simulink model "zumo_target"  (R2014a)
settings: Solver=ode3  SolverMode=SingleTasking  StartTime=0.0  StopTime=10  RelTol=1e-3
model workspace (MAT data in the model file):
  axleLength = Simulink.Parameter
  axleLength.Value = 9.5
  axleLength.Description = 'Distance between tire contact points
    | of the two wheels/treads
    | in units of centimeters.'
  axleLength.DataType = 'auto'
  commandPercmPerSecond = Simulink.Parameter
  commandPercmPerSecond.Value = 3.9547
  commandPercmPerSecond.Description = 'Convert units of ''command'' 
    | to units of ''cm/s''.
    | 
    | ''command'' is a value in the range [-256, 255].'
  commandPercmPerSecond.DataType = 'auto'
  symmetrizeMotors = Simulink.Parameter
  symmetrizeMotors.Value = 1
  symmetrizeMotors.Description = 'Scale one of the motor commands down 
    | (not up) to balance the motors. 
    | Once balanced, a value of x sent to either
    | motor will produce the same rate of rotation
    | in both motors.'
  symmetrizeMotors.DataType = 'auto'
  sampleTime = Simulink.Parameter
  sampleTime.Value = 0.01
  sampleTime.Description = 'Sample time (in seconds) of the trajectory simulator.'
  sampleTime.DataType = 'auto'
  commandThreshold = Simulink.Parameter
  commandThreshold.Value = 31.875
  commandThreshold.DataType = 'auto'
  plotRange = Simulink.Parameter
  plotRange.Value = 50
  plotRange.Description = 'Range of trajectory plot in units
    | of centimeters.'
  plotRange.DataType = 'auto'
undefined symbols (not defined in the file or in its folder): DiscIntNeverNeededParam
libraries: arduinolib x1, simulink x1, ZumoBotLib x1
settings Model: ExtModeTrigDuration=2  Creator=nrattner  LastModifiedBy=sandip
settings OptimizationCC: OptimizeModelRefInitCode=on  LifeSpan=1
settings DebuggingCC: UnderspecifiedInitializationDetection=Classic  SolverPrmCheckMsg=none
settings HardwareCC: ProdBitPerInt=16  ProdBitPerPointer=8  ProdIntDivRoundTo=Zero  ProdEndianess=LittleEndian  ProdWordSize=8  ProdHWDeviceType=Atmel->AVR
settings RTWCC: SystemTargetFile=realtime.tlc  GenerateMakefile=off  TemplateMakefile=realtime.tmf  Description=Run on Target Hardware  RTWVerbose=off  ProcessScript=realtime_make_rtw_hook
settings STFCustomTargetCC: TargetLibSuffix=.a  GenerateSampleERTMain=on  ConcurrentExecutionCompliant=off  GeneratePreprocessorConditionals=Use local settings  ERTCustomFileBanners=on  SupportNonInlinedSFcns=off  SupportVariableSizeSignals=on  MATLABClassNameForMDSCustomization=Simulink.SoftwareTarget.ERTCustomization  GRTInterface=off  SystemTargetFile=realtime.tlc
settings ERTTargetCC: CombineOutputUpdateFcns=off  SupportContinuousTime=on  SupportVariableSizeSignals=on  ExtModeTransport=3  ExtModeMexFile=ext_serial_win32_comm  ExtModeMexArgs=0 1 9600  ERTSrcFileBannerTemplate=realtime_code_template.cgt  ERTHdrFileBannerTemplate=realtime_code_template.cgt  ERTDataSrcFileTemplate=realtime_code_template.cgt  ERTDataHdrFileTemplate=realtime_code_template.cgt  ERTCustomFileTemplate=realtime_file_process.tlc

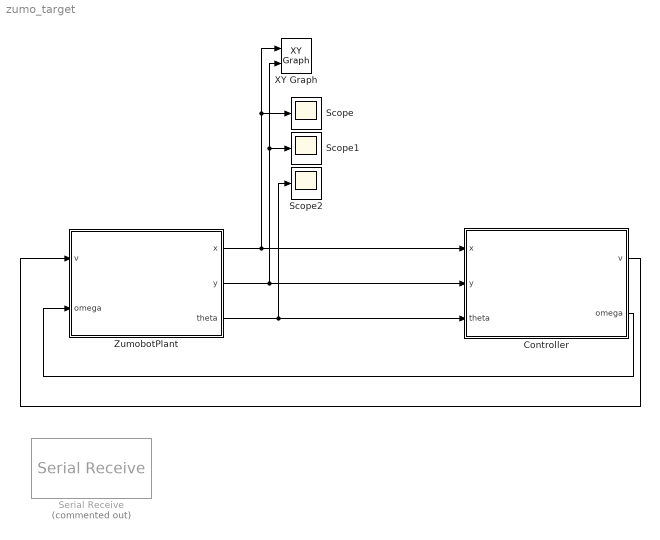
== system zumo_target ==
  Controller : Subsystem
  Scope : Scope
      settings: YMin=-0.000967084  YMax=-0.000967084
  Scope1 : Scope
      settings: YMin=0.0106562  YMax=0.0106562
  Scope2 : Scope
      settings: YMin=1.6613  YMax=1.6613  SaveName=ScopeData2
  Serial Receive : arduinolib/Serial Receive  Commented=on  portNumber=0  showOutStatus=on  sampleTime=1e-3
  XY Graph : simulink/Sinks/XY Graph  xmin=-10  xmax=10  ymin=-10  ymax=10  st=-1
  ZumobotPlant : Subsystem  Variant=on
  wires:
  ZumobotPlant/1(x) -> XY Graph/1, Scope/1, Controller/1(x)
  ZumobotPlant/2(y) -> Controller/2(y), XY Graph/2, Scope1/1
  ZumobotPlant/3(theta) -> Controller/3(theta), Scope2/1
  Controller/1(v) -> ZumobotPlant/1(v)
  Controller/2(omega) -> ZumobotPlant/2(omega)

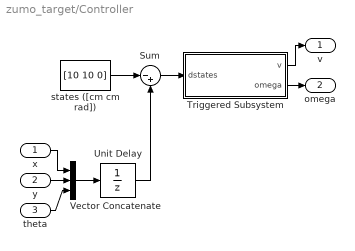
== system zumo_target/Controller ==
  x : Inport
  y : Inport  Port=2
  theta : Inport  Port=3
  Sum : Sum  Inputs=|-+
  Triggered Subsystem : Subsystem  TreatAsAtomicUnit=on
  Unit Delay : UnitDelay  SampleTime=-1
  Vector Concatenate : Concatenate  NumInputs=3
  states ([cm cm rad]) : Constant  Value=[10 10 0]
  v : Outport
  omega : Outport  Port=2
  wires:
  Unit Delay/1 -> Sum/2
  Vector Concatenate/1 -> Unit Delay/1
  Sum/1 -> Triggered Subsystem/1(dstates)
  states ([cm cm rad])/1 -> Sum/1
  Triggered Subsystem/1(v) -> v/1
  Triggered Subsystem/2(omega) -> omega/1
  y/1 -> Vector Concatenate/2
  theta/1 -> Vector Concatenate/3
  x/1 -> Vector Concatenate/1

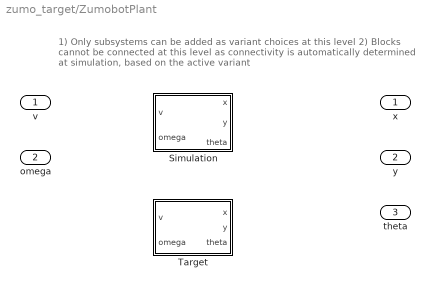
== system zumo_target/ZumobotPlant ==
  note: 1) Only subsystems can be added as variant choices at this level
      | 2) Blocks cannot be connected at this level as connectivity is
      | automatically determined at simulation, based on the active variant
  v : Inport
  omega : Inport  Port=2
  Simulation : Subsystem  VariantControl=sim==1
  Target : Subsystem  VariantControl=sim==0
  x : Outport
  y : Outport  Port=2
  theta : Outport  Port=3

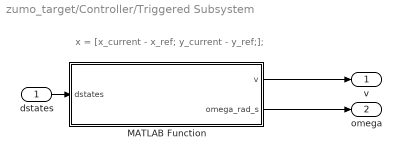
== system zumo_target/Controller/Triggered Subsystem ==
  note: x = [x_current - x_ref; y_current - y_ref;];
  dstates : Inport
  MATLAB Function : MATLAB Function  TreatAsAtomicUnit=on
  v : Outport
  omega : Outport  Port=2
  wires:
  dstates/1 -> MATLAB Function/1(dstates)
  MATLAB Function/1(v) -> v/1
  MATLAB Function/2(omega_rad_s) -> omega/1

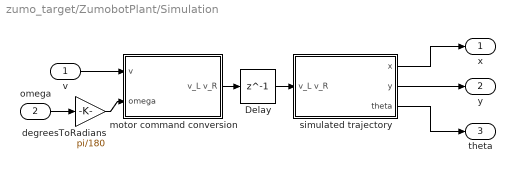
== system zumo_target/ZumobotPlant/Simulation ==
  v : Inport
  omega : Inport  Port=2
  Delay : Delay  DelayLength=1  InitialCondition=0
  degreesToRadians : Gain  Gain=pi/180
  motor command conversion : Subsystem
  simulated trajectory : Subsystem
  x : Outport
  y : Outport  Port=2
  theta : Outport  Port=3
  wires:
  v/1 -> motor command conversion/1(v)
  simulated trajectory/1(x) -> x/1
  simulated trajectory/2(y) -> y/1
  omega/1 -> degreesToRadians/1
  simulated trajectory/3(theta) -> theta/1
  degreesToRadians/1 -> motor command conversion/2(omega)
  motor command conversion/1(v_L v_R) -> Delay/1
  Delay/1 -> simulated trajectory/1(v_L v_R)

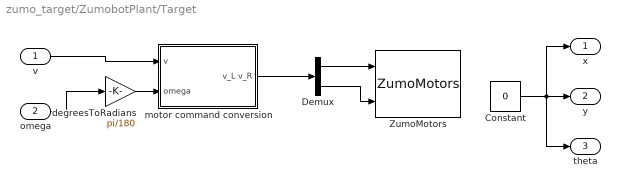
== system zumo_target/ZumobotPlant/Target ==
  v : Inport
  omega : Inport  Port=2
  Constant : Constant  Value=0
  Demux : Demux  Outputs=2
  ZumoMotors : ZumoBotLib/ZumoMotors  flipLeft=off  flipRight=off
  degreesToRadians : Gain  Gain=pi/180
  motor command conversion : Subsystem
  x : Outport
  y : Outport  Port=2
  theta : Outport  Port=3
  wires:
  motor command conversion/1(v_L v_R) -> Demux/1
  Demux/1 -> ZumoMotors/1
  Demux/2 -> ZumoMotors/2
  v/1 -> motor command conversion/1(v)
  Constant/1 -> theta/1, x/1, y/1
  omega/1 -> degreesToRadians/1
  degreesToRadians/1 -> motor command conversion/2(omega)

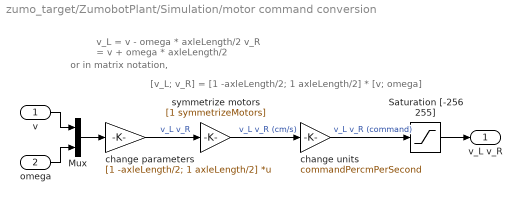
== system zumo_target/ZumobotPlant/Simulation/motor command conversion ==
  note: or in matrix notation,
  note: v_L  = v - omega * axleLength/2
      | v_R = v + omega * axleLength/2
  note: [v_L; v_R] = [1 -axleLength/2; 1 axleLength/2] * [v; omega]
  v : Inport
  omega : Inport  Port=2
  Mux : Mux  Inputs=2
  Saturation [-256 255] : Saturate  UpperLimit=255  LowerLimit=-256
  change parameters : Gain  Gain=[1 -axleLength/2; 1 axleLength/2]  Multiplication=Matrix(K*u)
  change units : Gain  Gain=commandPercmPerSecond
  symmetrize motors : Gain  Gain=[1 symmetrizeMotors]
  v_L v_R : Outport
  wires:
  change parameters/1 -> symmetrize motors/1  "v_L v_R"
  change units/1 -> Saturation [-256 255]/1  "v_L v_R (command)"
  symmetrize motors/1 -> change units/1  "v_L v_R (cm/s)"
  Saturation [-256 255]/1 -> v_L v_R/1
  Mux/1 -> change parameters/1
  omega/1 -> Mux/2
  v/1 -> Mux/1

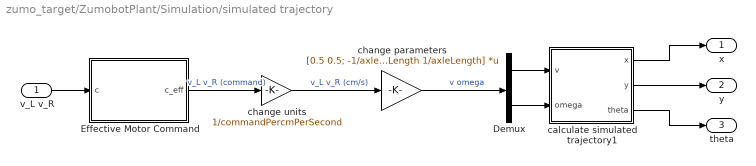
== system zumo_target/ZumobotPlant/Simulation/simulated trajectory ==
  v_L v_R : Inport
  Demux : Demux  Outputs=2
  Effective Motor Command : Subsystem
  calculate simulated trajectory1 : Subsystem
  change parameters : Gain  Gain=[0.5 0.5; -1/axleLength 1/axleLength]  Multiplication=Matrix(K*u)
  change units : Gain  Gain=1/commandPercmPerSecond
  x : Outport
  y : Outport  Port=2
  theta : Outport  Port=3
  wires:
  Demux/2 -> calculate simulated trajectory1/2(omega)
  Demux/1 -> calculate simulated trajectory1/1(v)
  v_L v_R/1 -> Effective Motor Command/1(c)
  Effective Motor Command/1(c_eff) -> change units/1  "v_L v_R (command)"
  change units/1 -> change parameters/1  "v_L v_R (cm/s)"
  change parameters/1 -> Demux/1  "v omega"
  calculate simulated trajectory1/2(y) -> y/1
  calculate simulated trajectory1/3(theta) -> theta/1
  calculate simulated trajectory1/1(x) -> x/1

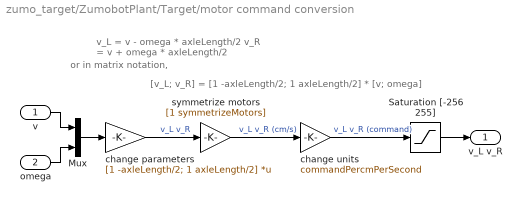
== system zumo_target/ZumobotPlant/Target/motor command conversion ==
  note: or in matrix notation,
  note: v_L  = v - omega * axleLength/2
      | v_R = v + omega * axleLength/2
  note: [v_L; v_R] = [1 -axleLength/2; 1 axleLength/2] * [v; omega]
  v : Inport
  omega : Inport  Port=2
  Mux : Mux  Inputs=2
  Saturation [-256 255] : Saturate  UpperLimit=255  LowerLimit=-256
  change parameters : Gain  Gain=[1 -axleLength/2; 1 axleLength/2]  Multiplication=Matrix(K*u)
  change units : Gain  Gain=commandPercmPerSecond
  symmetrize motors : Gain  Gain=[1 symmetrizeMotors]
  v_L v_R : Outport
  wires:
  change parameters/1 -> symmetrize motors/1  "v_L v_R"
  change units/1 -> Saturation [-256 255]/1  "v_L v_R (command)"
  symmetrize motors/1 -> change units/1  "v_L v_R (cm/s)"
  Saturation [-256 255]/1 -> v_L v_R/1
  Mux/1 -> change parameters/1
  omega/1 -> Mux/2
  v/1 -> Mux/1

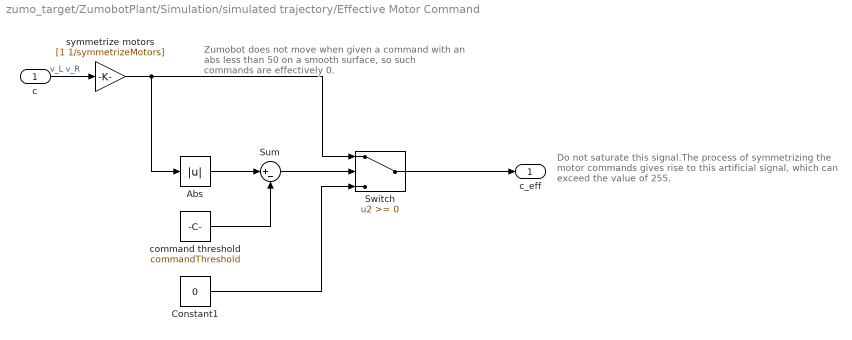
== system zumo_target/ZumobotPlant/Simulation/simulated trajectory/Effective Motor Command ==
  note: Zumobot does not move when given a command
      | with an abs less than 50 on a smooth surface,
      | so such commands are effectively 0.
  note: Do not saturate this signal.The process of symmetrizing
      | the motor commands gives rise to this artificial signal,
      | which can exceed the value of 255.
  c : Inport
  Abs : Abs
  Constant1 : Constant  Value=0
  Sum : Sum  Inputs=|+-
  Switch : Switch
  command threshold : Constant  Value=commandThreshold
  symmetrize motors : Gain  Gain=[1 1/symmetrizeMotors]
  c_eff : Outport
  wires:
  Switch/1 -> c_eff/1
  symmetrize motors/1 -> Abs/1, Switch/1
  Sum/1 -> Switch/2
  Abs/1 -> Sum/1
  command threshold/1 -> Sum/2
  c/1 -> symmetrize motors/1  "v_L v_R"
  Constant1/1 -> Switch/3

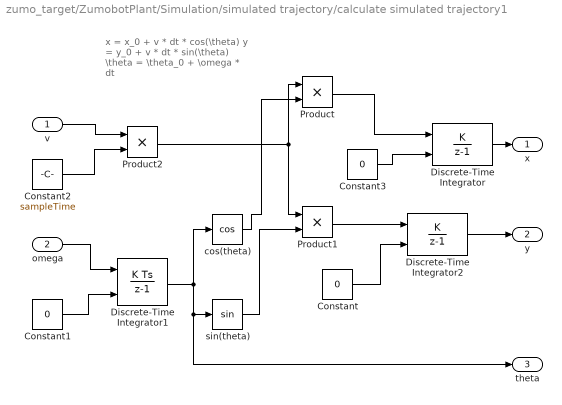
== system zumo_target/ZumobotPlant/Simulation/simulated trajectory/calculate simulated trajectory1 ==
  note: x = x_0 + v * dt * cos(\theta)
      | y = y_0 + v * dt * sin(\theta)
      | \theta = \theta_0 + \omega * dt
  v : Inport
  omega : Inport  Port=2
  Constant : Constant  Value=0
  Constant1 : Constant  Value=0
  Constant2 : Constant  Value=sampleTime
  Constant3 : Constant  Value=0
  Discrete-Time Integrator : DiscreteIntegrator  IntegratorMethod=Accumulation: Forward Euler  InitialConditionSource=external  InitialConditionSetting=State (most efficient)  SampleTime=-1  ICPrevOutput=DiscIntNeverNeededParam  ICPrevScaledInput=DiscIntNeverNeededParam
  Discrete-Time Integrator1 : DiscreteIntegrator  InitialConditionSource=external  SampleTime=-1  ICPrevOutput=DiscIntNeverNeededParam  ICPrevScaledInput=DiscIntNeverNeededParam
  Discrete-Time Integrator2 : DiscreteIntegrator  IntegratorMethod=Accumulation: Forward Euler  InitialConditionSource=external  InitialConditionSetting=State (most efficient)  SampleTime=-1  ICPrevOutput=DiscIntNeverNeededParam  ICPrevScaledInput=DiscIntNeverNeededParam
  Product : Product
  Product1 : Product
  Product2 : Product
  cos(theta) : Trigonometry  Operator=cos
  sin(theta) : Trigonometry
  x : Outport
  y : Outport  Port=2
  theta : Outport  Port=3
  wires:
  omega/1 -> Discrete-Time Integrator1/1
  v/1 -> Product2/1
  Discrete-Time Integrator1/1 -> theta/1, sin(theta)/1, cos(theta)/1
  Product/1 -> Discrete-Time Integrator/1
  cos(theta)/1 -> Product/2
  Product2/1 -> Product/1, Product1/1
  sin(theta)/1 -> Product1/2
  Constant3/1 -> Discrete-Time Integrator/2
  Constant1/1 -> Discrete-Time Integrator1/2
  Constant2/1 -> Product2/2
  Discrete-Time Integrator/1 -> x/1
  Product1/1 -> Discrete-Time Integrator2/1
  Discrete-Time Integrator2/1 -> y/1
  Constant/1 -> Discrete-Time Integrator2/2

== matlab function zumo_target/Controller/Triggered Subsystem/MATLAB Function ==
  data: dstates input; v output; omega_rad_s output
function [v, omega_rad_s] = minion_limitCycle3(dstates)
%#codegen
% This function expects the dstates to be the difference of 
% dx = x_curr - x_dest; dy = y_curr - y_dest; dth = th_curr - th_dest;

dx = dstates(1);% cm
dy = dstates(2);% cm
dth = dstates(3);% rad

min_res = 1; %cm
kp1 = 2;
kp2 = 12;
kd1 = 3;
kd2 = 7;
dt = 0.01;

if norm([dx dy]) < min_res
    % its converged, hence early return and force the robot to stop
    v = 0;
    omega_rad_s = 0;
    disp('Returning early as converged');
    return;
end
%% 
cth = cos(dth);
sth = sin(dth);

%% region division
region = 0; % initialize region
if dx >= 0 && dy >= 0     % add
    region = 1;
elseif dx < 0 && dy >= 0  % sugar
    region = 2;
elseif dx < 0 && dy < 0   % to
    region = 3;
elseif dx >= 0 && dy < 0  % coffee
    region = 4;
else
    error('Bad region: should not be here.');
end
%% region based inputs
if region == 2 || region == 3
    v = 10;
else % region = 1 || 4
    v = -10;
end
%% computing v and omega 
xd = v*cth;
yd = v*sth;

u1 = -kp1*dx - kd1*xd;
u2 = -kp2*dy - kd2*yd;

zeta_dot = u1*cth + u2*sth;
zeta = zeta_dot * dt;

% v = v + zeta; % cm/s
omega_rad_s = (u2*cth - u1*cth)/zeta; %rad/s
% maximum omega(rad/s) allowed = ~2*pi/sec
if omega_rad_s > 2*pi
    omega_rad_s = 2*pi;
elseif omega_rad_s < -2*pi
    omega_rad_s = -2*pi;
end
% convert rad/s into deg/s (as the plant model accepts that)
omega = omega_rad_s * (180/(2*pi));
[v omega]
